simulink model "Decouverte_Poster"  (R2022a)
settings: Solver=VariableStepAuto  StartTime=0.0  StopTime=inf  RelTol=1e-3
libraries: fl_lib x10, nesl_utility x3
settings Model: Creator=xavier.pessoles2  LastModifiedBy=xavier.pessoles2
settings DebuggingCC: UnconnectedInputMsg=warning  UnconnectedOutputMsg=warning  UnconnectedLineMsg=warning
settings RTWCC: DLArmComputeVersion=19.05

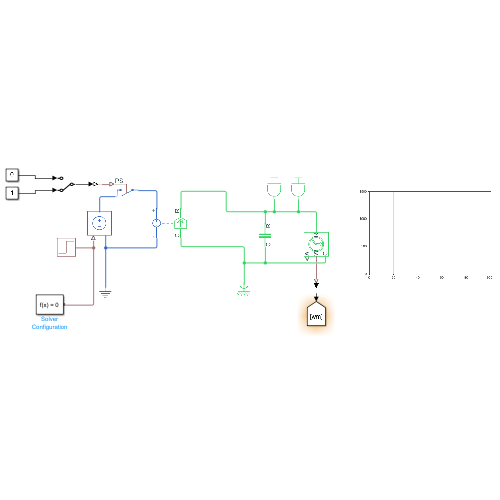
[thumbnail: Simulink's stored preview of the top-level diagram]
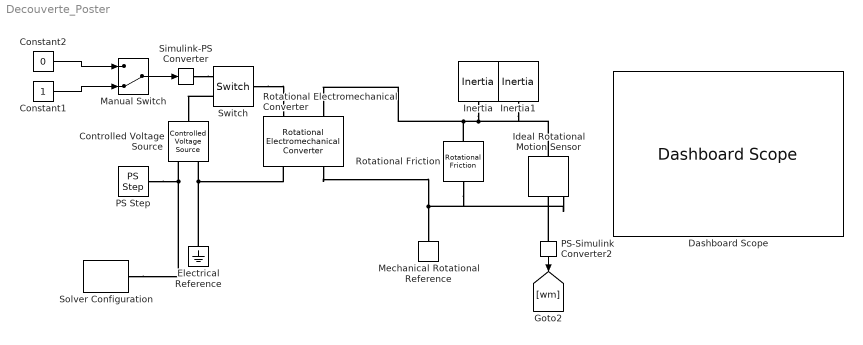
== system Decouverte_Poster ==
  Constant1 : Constant
  Constant2 : Constant  Value=0
  Controlled Voltage Source : fl_lib/Electrical/Electrical Sources/Controlled Voltage Source
      settings: SourceProductBaseCode=PW,SS,VE
  Dashboard Scope : DashboardScope  Ymin=0  Ymax=1500  ScaleAtStop=off
  Electrical Reference : fl_lib/Electrical/Electrical Elements/Electrical Reference
      settings: SourceProductBaseCode=PW,SS,VE
  Ideal Rotational Motion Sensor : fl_lib/Mechanical/Mechanical Sensors/Ideal Rotational Motion Sensor  wrap_angle=simscape.enum.onoff.off  offset=0 rad
      settings: SourceProductBaseCode=PW,SS,VE
  Inertia : fl_lib/Mechanical/Rotational Elements/Inertia  inertia=3e-6 kg*m^2  num_ports=foundation.enum.numPorts2.one  w_specify=off  w_priority=High  w=0 rad/s  w_nominal_specify=off  w_nominal_unit=rad/s  w_nominal_value=1  t_specify=off  t_priority=None  t=0 N*m  t_nominal_specify=off  t_nominal_unit=N*m  t_nominal_value=1
      settings: SourceProductBaseCode=PW,SS,VE
  Inertia1 : fl_lib/Mechanical/Rotational Elements/Inertia  inertia=1e-5 kg*m^2  num_ports=foundation.enum.numPorts2.one  w_specify=off  w_priority=High  w=0 rad/s  w_nominal_specify=off  w_nominal_unit=rad/s  w_nominal_value=1  t_specify=off  t_priority=None  t=0 N*m  t_nominal_specify=off  t_nominal_unit=N*m  t_nominal_value=1
      settings: SourceProductBaseCode=PW,SS,VE
  Manual Switch : ManualSwitch  CurrentSetting=0
  Mechanical Rotational Reference : fl_lib/Mechanical/Rotational Elements/Mechanical Rotational Reference
      settings: SourceProductBaseCode=PW,SS,VE
  PS Step : fl_lib/Physical Signals/Sources/PS Step  step_time=0 s  initial_value=0  final_value=12
      settings: SourceProductBaseCode=PW,SS,VE
  PS-Simulink Converter2 : nesl_utility/PS-Simulink Converter  PhysicalDomain=network_engine_domain  SubClassName=ps_output  LeftPortType=input  RightPortType=output  PseudoPeriodic=off  Frequencies=[]  VectorFormat=1-D array  Unit=inherit  AffineConversion=off
      settings: SourceProductBaseCode=SS,PW,VE
  Rotational Electromechanical Converter : fl_lib/Electrical/Electrical Elements/Rotational Electromechanical Converter  K=0.009 V*s/rad  i_specify=off  i_priority=None  i=0 A  i_nominal_specify=off  i_nominal_unit=A  i_nominal_value=1  v_specify=off  v_priority=None  v=0 V  v_nominal_specify=off  v_nominal_unit=V  v_nominal_value=1  t_specify=off  t_priority=None  t=0 N*m  t_nominal_specify=off  t_nominal_unit=N*m  t_nominal_value=1  w_specify=off  w_priority=None  w=0 rad/s  w_nominal_specify=off  w_nominal_unit=rad/s  w_nominal_value=1
      settings: SourceProductBaseCode=PW,SS,VE
  Rotational Friction : fl_lib/Mechanical/Rotational Elements/Rotational Friction  brkwy_trq=0.0000000001 N*m  brkwy_vel=0.0000000001 rad/s  Col_trq=0.0000000001 N*m  visc_coef=0.000025 N*m/(rad/s)  w_specify=off  w_priority=None  w=0 rad/s  w_nominal_specify=off  w_nominal_unit=rad/s  w_nominal_value=1  t_specify=off  t_priority=None  t=0 N*m  t_nominal_specify=off  t_nominal_unit=N*m  t_nominal_value=1
      settings: SourceProductBaseCode=PW,SS,VE
  Simulink-PS Converter : nesl_utility/Simulink-PS Converter  PhysicalDomain=network_engine_domain  SubClassName=ps_input  LeftPortType=input  RightPortType=output  PseudoPeriodic=off  Frequencies=[]  NoiseDistribution=none  NoiseParameters=[]  Unit=1  AffineConversion=off  FilteringAndDerivatives=provide  SimscapeFilterOrder=1  InputFilterTimeConstant=0.001  UdotUserProvided=0
      settings: SourceProductBaseCode=SS,PW,VE
  Solver Configuration : nesl_utility/Solver Configuration  PhysicalDomain=network_engine_domain  SubClassName=solver  LeftPortType=input  RightPortType=generic  Tones=[]  Harmonics=[]  SimulateNoise=off  Profile=off  UseLocalSampling=off  EnableSwitchedLinearOptims=on  FrequencyDomain=off  UseCCode=off  RelTol=0.001  AbsTol=1e-06  MinStep=1e-09  ToWorkspace=off  RevertToSquareIcSolve=off  NumHomotopyIterations=100  PhasorMode=off  PhasorModeNumHarmonics=1  IndexReductionMethod=DerivativeReplacement  DoDC=off  ResidualTolerance=1e-09  UseLocalSolver=off  LocalSolverChoice=NE_BACKWARD_EULER_ADVANCER  LocalSolverSampleTime=0.001  DoFixedCost=off  MaxNonlinIter=3  MaxModeIter=2  ComputeImpulses=off  ImpulseIterations=2  LinearAlgebra=auto  LinearAlgebraNumThread=0  EquationFormulation=NE_TIME_EF  DelaysMemoryBudget=1024  AutomaticFiltering=on  FilteringTimeConstant=0.001  PartitionStorageMethod=AS_NEEDED  PartitionMemoryBudget=1024  PartitionMethod=ROBUST
      settings: SourceProductBaseCode=SS,PW,VE
  Switch : fl_lib/Electrical/Electrical Elements/Switch  R_closed=0.0001 Ohm  G_open=1e-8 1/Ohm  Threshold=0.5  i_specify=off  i_priority=None  i=0 A  i_nominal_specify=off  i_nominal_unit=A  i_nominal_value=1  v_specify=off  v_priority=None  v=0 V  v_nominal_specify=off  v_nominal_unit=V  v_nominal_value=1
      settings: SourceProductBaseCode=PW,SS,VE
  wires:
  PS-Simulink Converter2/1 -> [wm]
  Manual Switch/1 -> Simulink-PS Converter/1
  Constant2/1 -> Manual Switch/1
  Constant1/1 -> Manual Switch/2
  connections:
  PS Step/RConn1 -- Solver Configuration/RConn1 -- Controlled Voltage Source/RConn1
  Switch/LConn1 -- Rotational Electromechanical Converter/LConn1
  Switch/RConn2 -- Controlled Voltage Source/LConn1
  Rotational Electromechanical Converter/RConn2 -- Mechanical Rotational Reference/LConn1 -- Rotational Friction/RConn1 -- Ideal Rotational Motion Sensor/RConn1
  Inertia/LConn1 -- Inertia1/LConn1 -- Ideal Rotational Motion Sensor/LConn1 -- Rotational Electromechanical Converter/LConn2 -- Rotational Friction/LConn1
  Electrical Reference/LConn1 -- Controlled Voltage Source/RConn2 -- Rotational Electromechanical Converter/RConn1
  PS-Simulink Converter2/LConn1 -- Ideal Rotational Motion Sensor/RConn2
  Simulink-PS Converter/RConn1 -- Switch/RConn1
